simulink model "s_c_nbe_m32k"  (R2016b)
(part 2 of 104)

      mask prompts: io_dir "I/O direction"; io_delay "I/O delay"; init_val "Initial Value"; sample_period "Sample period"; names "Bitfield names [msb...lsb]"; bitwidths "Bitfield widths"; bin_pts "Bitfield binary pts"; arith_types "Bitfield types, ufix=0, fix=1, bool=2"; sim_port "Provide sim input/output?"; show_format "Print format string?"
      mask help: A 32-bit software-accessible register. Can be divided into bitfields of varying widths and types using the fields in the block mask.
      mask init:
      | swreg_init(gcb)
      settings: AttributesFormatString=1input:uf16.15 = 16 bits
      mask TypeOptions io_dir: To Processor | From Processor
      mask Callback io_dir:
      | mask_enables = get_param(gcb, 'MaskEnables');
      | mask_names = get_param(gcb, 'MaskNames');
      | if strcmp(get_param(gcb, 'io_dir'), 'To Processor'),
      |     mask_enables{ismember(mask_names, 'sample_period')} = 'off';
      | else
      |     mask_enables{ismember(mask_names, 'sample_period')} = 'on';
      | end
      | set_param(gcb, 'MaskEnables', mask_enables);
      mask DialogControl ParameterTabVar0 Prompt: Setup
  scale_p1_ddc0 : Subsystem  Tag=xps:sw_reg  AncestorBlock=xps_library/Memory/software_register  mask(swreg){io_dir=From Processor, io_delay=1, init_val=0, sample_period=1, names=scale, bitwidths=16, bin_pts=15, arith_types=0, sim_port=on, show_format=on}
      mask prompts: io_dir "I/O direction"; io_delay "I/O delay"; init_val "Initial Value"; sample_period "Sample period"; names "Bitfield names [msb...lsb]"; bitwidths "Bitfield widths"; bin_pts "Bitfield binary pts"; arith_types "Bitfield types, ufix=0, fix=1, bool=2"; sim_port "Provide sim input/output?"; show_format "Print format string?"
      mask help: A 32-bit software-accessible register. Can be divided into bitfields of varying widths and types using the fields in the block mask.
      mask init:
      | swreg_init(gcb)
      settings: AttributesFormatString=1input:uf16.15 = 16 bits
      mask TypeOptions io_dir: To Processor | From Processor
      mask Callback io_dir:
      | mask_enables = get_param(gcb, 'MaskEnables');
      | mask_names = get_param(gcb, 'MaskNames');
      | if strcmp(get_param(gcb, 'io_dir'), 'To Processor'),
      |     mask_enables{ismember(mask_names, 'sample_period')} = 'off';
      | else
      |     mask_enables{ismember(mask_names, 'sample_period')} = 'on';
      | end
      | set_param(gcb, 'MaskEnables', mask_enables);
      mask DialogControl ParameterTabVar0 Prompt: Setup
  sync_time_lsw : Subsystem  Tag=xps:sw_reg  AncestorBlock=xps_library/Memory/software_register  mask(swreg){io_dir=To Processor, io_delay=0, init_val=0, sample_period=1, names=reg, bitwidths=32, bin_pts=0, arith_types=0, sim_port=off, show_format=on}
      mask prompts: io_dir "I/O direction"; io_delay "I/O delay"; init_val "Initial Value"; sample_period "Sample period"; names "Bitfield names [msb...lsb]"; bitwidths "Bitfield widths"; bin_pts "Bitfield binary pts"; arith_types "Bitfield types, ufix=0, fix=1, bool=2"; sim_port "Provide sim input/output?"; show_format "Print format string?"
      mask help: A 32-bit software-accessible register. Can be divided into bitfields of varying widths and types using the fields in the block mask.
      mask init:
      | swreg_init(gcb)
      settings: AttributesFormatString=1output:uf32.0 = 32 bits
      mask TypeOptions io_dir: To Processor | From Processor
      mask Callback io_dir:
      | mask_enables = get_param(gcb, 'MaskEnables');
      | mask_names = get_param(gcb, 'MaskNames');
      | if strcmp(get_param(gcb, 'io_dir'), 'To Processor'),
      |     mask_enables{ismember(mask_names, 'sample_period')} = 'off';
      | else
      |     mask_enables{ismember(mask_names, 'sample_period')} = 'on';
      | end
      | set_param(gcb, 'MaskEnables', mask_enables);
      mask DialogControl ParameterTabVar0 Prompt: Setup
  sync_time_msw : Subsystem  Tag=xps:sw_reg  AncestorBlock=xps_library/Memory/software_register  mask(swreg){io_dir=To Processor, io_delay=0, init_val=0, sample_period=1, names=reg, bitwidths=16, bin_pts=0, arith_types=0, sim_port=off, show_format=on}
      mask prompts: io_dir "I/O direction"; io_delay "I/O delay"; init_val "Initial Value"; sample_period "Sample period"; names "Bitfield names [msb...lsb]"; bitwidths "Bitfield widths"; bin_pts "Bitfield binary pts"; arith_types "Bitfield types, ufix=0, fix=1, bool=2"; sim_port "Provide sim input/output?"; show_format "Print format string?"
      mask help: A 32-bit software-accessible register. Can be divided into bitfields of varying widths and types using the fields in the block mask.
      mask init:
      | swreg_init(gcb)
      settings: AttributesFormatString=1output:uf16.0 = 16 bits
      mask TypeOptions io_dir: To Processor | From Processor
      mask Callback io_dir:
      | mask_enables = get_param(gcb, 'MaskEnables');
      | mask_names = get_param(gcb, 'MaskNames');
      | if strcmp(get_param(gcb, 'io_dir'), 'To Processor'),
      |     mask_enables{ismember(mask_names, 'sample_period')} = 'off';
      | else
      |     mask_enables{ismember(mask_names, 'sample_period')} = 'on';
      | end
      | set_param(gcb, 'MaskEnables', mask_enables);
      mask DialogControl ParameterTabVar0 Prompt: Setup
  time_gen : Subsystem  mask{n_bits_period=fft_stages-1-2, n_bits_increment=0, n_bits_counter=48-fft_stages}
      mask prompts: n_bits_period "Period (2^?)"; n_bits_increment "Increment (2^?)"; n_bits_counter "Counter size (2^?)"
  time_gen1 : Subsystem  mask{n_bits_period=fft_stages-1-2-1+8, n_bits_increment=0, n_bits_counter=48-(fft_stages+8)}
      mask prompts: n_bits_period "Period (2^?)"; n_bits_increment "Increment (2^?)"; n_bits_counter "Counter size (2^?)"
  tl_cd0_control : Subsystem  Tag=xps:sw_reg  AncestorBlock=xps_library/Memory/software_register  mask(swreg){io_dir=From Processor, io_delay=0, init_val=0, sample_period=1, names=load_time_lsw, bitwidths=32, bin_pts=0, arith_types=0, sim_port=on, show_format=on}
      mask prompts: io_dir "I/O direction"; io_delay "I/O delay"; init_val "Initial Value"; sample_period "Sample period"; names "Bitfield names [msb...lsb]"; bitwidths "Bitfield widths"; bin_pts "Bitfield binary pts"; arith_types "Bitfield types, ufix=0, fix=1, bool=2"; sim_port "Provide sim input/output?"; show_format "Print format string?"
      mask help: A 32-bit software-accessible register. Can be divided into bitfields of varying widths and types using the fields in the block mask.
      mask init:
      | swreg_init(gcb)
      settings: AttributesFormatString=1input:uf32.0 = 32 bits
      mask TypeOptions io_dir: To Processor | From Processor
      mask Callback io_dir:
      | mask_enables = get_param(gcb, 'MaskEnables');
      | mask_names = get_param(gcb, 'MaskNames');
      | if strcmp(get_param(gcb, 'io_dir'), 'To Processor'),
      |     mask_enables{ismember(mask_names, 'sample_period')} = 'off';
      | else
      |     mask_enables{ismember(mask_names, 'sample_period')} = 'on';
      | end
      | set_param(gcb, 'MaskEnables', mask_enables);
      mask DialogControl ParameterTabVar0 Prompt: Setup
  tl_cd0_control0 : Subsystem  Tag=xps:sw_reg  AncestorBlock=xps_library/Memory/software_register  mask(swreg){io_dir=From Processor, io_delay=0, init_val=0, sample_period=1, names=[arm load_immediate load_time_msw], bitwidths=[1 1 16], bin_pts=[0 0 0], arith_types=[2 2 0], sim_port=on, show_format=on}
      mask prompts: io_dir "I/O direction"; io_delay "I/O delay"; init_val "Initial Value"; sample_period "Sample period"; names "Bitfield names [msb...lsb]"; bitwidths "Bitfield widths"; bin_pts "Bitfield binary pts"; arith_types "Bitfield types, ufix=0, fix=1, bool=2"; sim_port "Provide sim input/output?"; show_format "Print format string?"
      mask help: A 32-bit software-accessible register. Can be divided into bitfields of varying widths and types using the fields in the block mask.
      mask init:
      | swreg_init(gcb)
      settings: AttributesFormatString=3 inputs:b,b,uf16.0 = 18 bits
      mask TypeOptions io_dir: To Processor | From Processor
      mask Callback io_dir:
      | mask_enables = get_param(gcb, 'MaskEnables');
      | mask_names = get_param(gcb, 'MaskNames');
      | if strcmp(get_param(gcb, 'io_dir'), 'To Processor'),
      |     mask_enables{ismember(mask_names, 'sample_period')} = 'off';
      | else
      |     mask_enables{ismember(mask_names, 'sample_period')} = 'on';
      | end
      | set_param(gcb, 'MaskEnables', mask_enables);
      mask DialogControl ParameterTabVar0 Prompt: Setup
  tl_cd1_control : Subsystem  Tag=xps:sw_reg  AncestorBlock=xps_library/Memory/software_register  mask(swreg){io_dir=From Processor, io_delay=0, init_val=0, sample_period=1, names=load_time_lsw, bitwidths=32, bin_pts=0, arith_types=0, sim_port=on, show_format=on}
      mask prompts: io_dir "I/O direction"; io_delay "I/O delay"; init_val "Initial Value"; sample_period "Sample period"; names "Bitfield names [msb...lsb]"; bitwidths "Bitfield widths"; bin_pts "Bitfield binary pts"; arith_types "Bitfield types, ufix=0, fix=1, bool=2"; sim_port "Provide sim input/output?"; show_format "Print format string?"
      mask help: A 32-bit software-accessible register. Can be divided into bitfields of varying widths and types using the fields in the block mask.
      mask init:
      | swreg_init(gcb)
      settings: AttributesFormatString=1input:uf32.0 = 32 bits
      mask TypeOptions io_dir: To Processor | From Processor
      mask Callback io_dir:
      | mask_enables = get_param(gcb, 'MaskEnables');
      | mask_names = get_param(gcb, 'MaskNames');
      | if strcmp(get_param(gcb, 'io_dir'), 'To Processor'),
      |     mask_enables{ismember(mask_names, 'sample_period')} = 'off';
      | else
      |     mask_enables{ismember(mask_names, 'sample_period')} = 'on';
      | end
      | set_param(gcb, 'MaskEnables', mask_enables);
      mask DialogControl ParameterTabVar0 Prompt: Setup
  tl_cd1_control0 : Subsystem  Tag=xps:sw_reg  AncestorBlock=xps_library/Memory/software_register  mask(swreg){io_dir=From Processor, io_delay=0, init_val=0, sample_period=1, names=[arm load_immediate load_time_msw], bitwidths=[1 1 16], bin_pts=[0 0 0], arith_types=[2 2 0], sim_port=on, show_format=on}
      mask prompts: io_dir "I/O direction"; io_delay "I/O delay"; init_val "Initial Value"; sample_period "Sample period"; names "Bitfield names [msb...lsb]"; bitwidths "Bitfield widths"; bin_pts "Bitfield binary pts"; arith_types "Bitfield types, ufix=0, fix=1, bool=2"; sim_port "Provide sim input/output?"; show_format "Print format string?"
      mask help: A 32-bit software-accessible register. Can be divided into bitfields of varying widths and types using the fields in the block mask.
      mask init:
      | swreg_init(gcb)
      settings: AttributesFormatString=3 inputs:b,b,uf16.0 = 18 bits
      mask TypeOptions io_dir: To Processor | From Processor
      mask Callback io_dir:
      | mask_enables = get_param(gcb, 'MaskEnables');
      | mask_names = get_param(gcb, 'MaskNames');
      | if strcmp(get_param(gcb, 'io_dir'), 'To Processor'),
      |     mask_enables{ismember(mask_names, 'sample_period')} = 'off';
      | else
      |     mask_enables{ismember(mask_names, 'sample_period')} = 'on';
      | end
      | set_param(gcb, 'MaskEnables', mask_enables);
      mask DialogControl ParameterTabVar0 Prompt: Setup
  tl_fd0 : Subsystem  mask(timed_latch){n_bits_time=48-fft_stages, n_bits_quantization=fft_stages, n_bits_counters=4}
      mask prompts: n_bits_time "Number bits in time to compare"; n_bits_quantization "Time offset from lsb"; n_bits_counters "Bits in status counters"
      mask help:
      | Latches load_value when armed and current_time matches requested time.
      | current_time should be in ADC samples.
      mask init:
      | set_param([gcb,'/status'], 'bitwidths', mat2str([1, repmat(n_bits_counters, 1, 2)]));
      mask Help:
      | When armed, will latch new value when current time matches the time
      | specified. The input time should be in samples and mask settings allow
      | a portion of this to be compared to cater for quantization. Arm and latch
      | counts allow the current state, pending and missed latch events to be
      | determined.
  tl_fd1 : Subsystem  mask(timed_latch){n_bits_time=48-fft_stages, n_bits_quantization=fft_stages, n_bits_counters=4}
      mask prompts: n_bits_time "Number bits in time to compare"; n_bits_quantization "Time offset from lsb"; n_bits_counters "Bits in status counters"
      mask help:
      | Latches load_value when armed and current_time matches requested time.
      | current_time should be in ADC samples.
      mask init:
      | set_param([gcb,'/status'], 'bitwidths', mat2str([1, repmat(n_bits_counters, 1, 2)]));
      mask Help:
      | When armed, will latch new value when current time matches the time
      | specified. The input time should be in samples and mask settings allow
      | a portion of this to be compared to cater for quantization. Arm and latch
      | counts allow the current state, pending and missed latch events to be
      | determined.
  tvg : Subsystem
  tvg_tone_levels : Subsystem  Tag=xps:sw_reg  AncestorBlock=xps_library/Memory/software_register  mask(swreg){io_dir=From Processor, io_delay=0, init_val=0, sample_period=1, names=[p0r p0i p1r p1i], bitwidths=8, bin_pts=7, arith_types=1, sim_port=on, show_format=on}
      mask prompts: io_dir "I/O direction"; io_delay "I/O delay"; init_val "Initial Value"; sample_period "Sample period"; names "Bitfield names [msb...lsb]"; bitwidths "Bitfield widths"; bin_pts "Bitfield binary pts"; arith_types "Bitfield types, ufix=0, fix=1, bool=2"; sim_port "Provide sim input/output?"; show_format "Print format string?"
      mask help: A 32-bit software-accessible register. Can be divided into bitfields of varying widths and types using the fields in the block mask.
      mask init:
      | swreg_init(gcb)
      settings: AttributesFormatString=4 inputs:f8.7,f8.7,f8.7,f8.7 = 32 bits
      mask TypeOptions io_dir: To Processor | From Processor
      mask Callback io_dir:
      | mask_enables = get_param(gcb, 'MaskEnables');
      | mask_names = get_param(gcb, 'MaskNames');
      | if strcmp(get_param(gcb, 'io_dir'), 'To Processor'),
      |     mask_enables{ismember(mask_names, 'sample_period')} = 'off';
      | else
      |     mask_enables{ismember(mask_names, 'sample_period')} = 'on';
      | end
      | set_param(gcb, 'MaskEnables', mask_enables);
      mask DialogControl ParameterTabVar0 Prompt: Setup
  tvg_tone_targets : Subsystem  Tag=xps:sw_reg  AncestorBlock=xps_library/Memory/software_register  mask(swreg){io_dir=From Processor, io_delay=0, init_val=0, sample_period=1, names=[p0 p1], bitwidths=fft_stages, bin_pts=0, arith_types=0, sim_port=on, show_format=on}
      mask prompts: io_dir "I/O direction"; io_delay "I/O delay"; init_val "Initial Value"; sample_period "Sample period"; names "Bitfield names [msb...lsb]"; bitwidths "Bitfield widths"; bin_pts "Bitfield binary pts"; arith_types "Bitfield types, ufix=0, fix=1, bool=2"; sim_port "Provide sim input/output?"; show_format "Print format string?"
      mask help: A 32-bit software-accessible register. Can be divided into bitfields of varying widths and types using the fields in the block mask.
      mask init:
      | swreg_init(gcb)
      settings: AttributesFormatString=2 inputs:uf13.0,uf13.0 = 26 bits
      mask TypeOptions io_dir: To Processor | From Processor
      mask Callback io_dir:
      | mask_enables = get_param(gcb, 'MaskEnables');
      | mask_names = get_param(gcb, 'MaskNames');
      | if strcmp(get_param(gcb, 'io_dir'), 'To Processor'),
      |     mask_enables{ismember(mask_names, 'sample_period')} = 'off';
      | else
      |     mask_enables{ismember(mask_names, 'sample_period')} = 'on';
      | end
      | set_param(gcb, 'MaskEnables', mask_enables);
      mask DialogControl ParameterTabVar0 Prompt: Setup
  we_delay1 : Subsystem  AncestorBlock=casper_library_delays/pipeline  mask(pipeline){latency=2}
      mask help:
      | An explicitly laid-out delay line to avoid mapping to SRL16s
      | for use in pipelining to help achieve timing closure.
      mask init:
      | pipeline_init(gcb,'latency',latency);
      settings: AttributesFormatString=Latency = %<latency>
      mask Display:
      | port_label('input', 1, 'd');
      | port_label('output', 1, 'q');
      | disp(['Z^-', num2str(latency)]);
  we_delay112 : Subsystem  AncestorBlock=casper_library_delays/pipeline  mask(pipeline){latency=2}
      mask help:
      | An explicitly laid-out delay line to avoid mapping to SRL16s
      | for use in pipelining to help achieve timing closure.
      mask init:
      | pipeline_init(gcb,'latency',latency);
      settings: AttributesFormatString=Latency = %<latency>
      mask Display:
      | port_label('input', 1, 'd');
      | port_label('output', 1, 'q');
      | disp(['Z^-', num2str(latency)]);
  we_delay113 : Subsystem  AncestorBlock=casper_library_delays/pipeline  mask(pipeline){latency=2}
      mask help:
      | An explicitly laid-out delay line to avoid mapping to SRL16s
      | for use in pipelining to help achieve timing closure.
      mask init:
      | pipeline_init(gcb,'latency',latency);
      settings: AttributesFormatString=Latency = %<latency>
      mask Display:
      | port_label('input', 1, 'd');
      | port_label('output', 1, 'q');
      | disp(['Z^-', num2str(latency)]);
  we_delay114 : Subsystem  AncestorBlock=casper_library_delays/pipeline  mask(pipeline){latency=2}
      mask help:
      | An explicitly laid-out delay line to avoid mapping to SRL16s
      | for use in pipelining to help achieve timing closure.
      mask init:
      | pipeline_init(gcb,'latency',latency);
      settings: AttributesFormatString=Latency = %<latency>
      mask Display:
      | port_label('input', 1, 'd');
      | port_label('output', 1, 'q');
      | disp(['Z^-', num2str(latency)]);
  we_delay115 : Subsystem  AncestorBlock=casper_library_delays/pipeline  mask(pipeline){latency=2}
      mask help:
      | An explicitly laid-out delay line to avoid mapping to SRL16s
      | for use in pipelining to help achieve timing closure.
      mask init:
      | pipeline_init(gcb,'latency',latency);
      settings: AttributesFormatString=Latency = %<latency>
      mask Display:
      | port_label('input', 1, 'd');
      | port_label('output', 1, 'q');
      | disp(['Z^-', num2str(latency)]);
  we_delay116 : Subsystem  AncestorBlock=casper_library_delays/pipeline  mask(pipeline){latency=2}
      mask help:
      | An explicitly laid-out delay line to avoid mapping to SRL16s
      | for use in pipelining to help achieve timing closure.
      mask init:
      | pipeline_init(gcb,'latency',latency);
      settings: AttributesFormatString=Latency = %<latency>
      mask Display:
      | port_label('input', 1, 'd');
      | port_label('output', 1, 'q');
      | disp(['Z^-', num2str(latency)]);
  we_delay117 : Subsystem  AncestorBlock=casper_library_delays/pipeline  mask(pipeline){latency=2}
      mask help:
      | An explicitly laid-out delay line to avoid mapping to SRL16s
      | for use in pipelining to help achieve timing closure.
      mask init:
      | pipeline_init(gcb,'latency',latency);
      settings: AttributesFormatString=Latency = %<latency>
      mask Display:
      | port_label('input', 1, 'd');
      | port_label('output', 1, 'q');
      | disp(['Z^-', num2str(latency)]);
  we_delay124 : Subsystem  AncestorBlock=casper_library_delays/pipeline  mask(pipeline){latency=2}
      mask help:
      | An explicitly laid-out delay line to avoid mapping to SRL16s
      | for use in pipelining to help achieve timing closure.
      mask init:
      | pipeline_init(gcb,'latency',latency);
      settings: AttributesFormatString=Latency = %<latency>
      mask Display:
      | port_label('input', 1, 'd');
      | port_label('output', 1, 'q');
      | disp(['Z^-', num2str(latency)]);
  we_delay126 : Subsystem  AncestorBlock=casper_library_delays/pipeline  mask(pipeline){latency=2}
      mask help:
      | An explicitly laid-out delay line to avoid mapping to SRL16s
      | for use in pipelining to help achieve timing closure.
      mask init:
      | pipeline_init(gcb,'latency',latency);
      settings: AttributesFormatString=Latency = %<latency>
      mask Display:
      | port_label('input', 1, 'd');
      | port_label('output', 1, 'q');
      | disp(['Z^-', num2str(latency)]);
  we_delay13 : Subsystem  AncestorBlock=casper_library_delays/pipeline  mask(pipeline){latency=2}
      mask help:
      | An explicitly laid-out delay line to avoid mapping to SRL16s
      | for use in pipelining to help achieve timing closure.
      mask init:
      | pipeline_init(gcb,'latency',latency);
      settings: AttributesFormatString=Latency = %<latency>
      mask Display:
      | port_label('input', 1, 'd');
      | port_label('output', 1, 'q');
      | disp(['Z^-', num2str(latency)]);
  we_delay2 : Subsystem  AncestorBlock=casper_library_delays/pipeline  mask(pipeline){latency=2}
      mask help:
      | An explicitly laid-out delay line to avoid mapping to SRL16s
      | for use in pipelining to help achieve timing closure.
      mask init:
      | pipeline_init(gcb,'latency',latency);
      settings: AttributesFormatString=Latency = %<latency>
      mask Display:
      | port_label('input', 1, 'd');
      | port_label('output', 1, 'q');
      | disp(['Z^-', num2str(latency)]);
  we_delay29 : Subsystem  AncestorBlock=casper_library_delays/pipeline  mask(pipeline){latency=2}
      mask help:
      | An explicitly laid-out delay line to avoid mapping to SRL16s
      | for use in pipelining to help achieve timing closure.
      mask init:
      | pipeline_init(gcb,'latency',latency);
      settings: AttributesFormatString=Latency = %<latency>
      mask Display:
      | port_label('input', 1, 'd');
      | port_label('output', 1, 'q');
      | disp(['Z^-', num2str(latency)]);
  we_delay37 : Subsystem  AncestorBlock=casper_library_delays/pipeline  mask(pipeline){latency=2}
      mask help:
      | An explicitly laid-out delay line to avoid mapping to SRL16s
      | for use in pipelining to help achieve timing closure.
      mask init:
      | pipeline_init(gcb,'latency',latency);
      settings: AttributesFormatString=Latency = %<latency>
      mask Display:
      | port_label('input', 1, 'd');
      | port_label('output', 1, 'q');
      | disp(['Z^-', num2str(latency)]);
  we_delay38 : Subsystem  AncestorBlock=casper_library_delays/pipeline  mask(pipeline){latency=2}
      mask help:
      | An explicitly laid-out delay line to avoid mapping to SRL16s
      | for use in pipelining to help achieve timing closure.
      mask init:
      | pipeline_init(gcb,'latency',latency);
      settings: AttributesFormatString=Latency = %<latency>
      mask Display:
      | port_label('input', 1, 'd');
      | port_label('output', 1, 'q');
      | disp(['Z^-', num2str(latency)]);
  we_delay39 : Subsystem  AncestorBlock=casper_library_delays/pipeline  mask(pipeline){latency=2}
      mask help:
      | An explicitly laid-out delay line to avoid mapping to SRL16s
      | for use in pipelining to help achieve timing closure.
      mask init:
      | pipeline_init(gcb,'latency',latency);
      settings: AttributesFormatString=Latency = %<latency>
      mask Display:
      | port_label('input', 1, 'd');
      | port_label('output', 1, 'q');
      | disp(['Z^-', num2str(latency)]);
  we_delay41 : Subsystem  AncestorBlock=casper_library_delays/pipeline  mask(pipeline){latency=2}
      mask help:
      | An explicitly laid-out delay line to avoid mapping to SRL16s
      | for use in pipelining to help achieve timing closure.
      mask init:
      | pipeline_init(gcb,'latency',latency);
      settings: AttributesFormatString=Latency = %<latency>
      mask Display:
      | port_label('input', 1, 'd');
      | port_label('output', 1, 'q');
      | disp(['Z^-', num2str(latency)]);
  we_delay47 : Subsystem  AncestorBlock=casper_library_delays/pipeline  mask(pipeline){latency=2}
      mask help:
      | An explicitly laid-out delay line to avoid mapping to SRL16s
      | for use in pipelining to help achieve timing closure.
      mask init:
      | pipeline_init(gcb,'latency',latency);
      settings: AttributesFormatString=Latency = %<latency>
      mask Display:
      | port_label('input', 1, 'd');
      | port_label('output', 1, 'q');
      | disp(['Z^-', num2str(latency)]);
  we_delay48 : Subsystem  AncestorBlock=casper_library_delays/pipeline  mask(pipeline){latency=2}
      mask help:
      | An explicitly laid-out delay line to avoid mapping to SRL16s
      | for use in pipelining to help achieve timing closure.
      mask init:
      | pipeline_init(gcb,'latency',latency);
      settings: AttributesFormatString=Latency = %<latency>
      mask Display:
      | port_label('input', 1, 'd');
      | port_label('output', 1, 'q');
      | disp(['Z^-', num2str(latency)]);
  we_delay49 : Subsystem  AncestorBlock=casper_library_delays/pipeline  mask(pipeline){latency=2}
      mask help:
      | An explicitly laid-out delay line to avoid mapping to SRL16s
      | for use in pipelining to help achieve timing closure.
      mask init:
      | pipeline_init(gcb,'latency',latency);
      settings: AttributesFormatString=Latency = %<latency>
      mask Display:
      | port_label('input', 1, 'd');
      | port_label('output', 1, 'q');
      | disp(['Z^-', num2str(latency)]);
  we_delay50 : Subsystem  AncestorBlock=casper_library_delays/pipeline  mask(pipeline){latency=2}
      mask help:
      | An explicitly laid-out delay line to avoid mapping to SRL16s
      | for use in pipelining to help achieve timing closure.
      mask init:
      | pipeline_init(gcb,'latency',latency);
      settings: AttributesFormatString=Latency = %<latency>
      mask Display:
      | port_label('input', 1, 'd');
      | port_label('output', 1, 'q');
      | disp(['Z^-', num2str(latency)]);
  we_delay7 : Subsystem  AncestorBlock=casper_library_delays/pipeline  mask(pipeline){latency=2}
      mask help:
      | An explicitly laid-out delay line to avoid mapping to SRL16s
      | for use in pipelining to help achieve timing closure.
      mask init:
      | pipeline_init(gcb,'latency',latency);
      settings: AttributesFormatString=Latency = %<latency>
      mask Display:
      | port_label('input', 1, 'd');
      | port_label('output', 1, 'q');
      | disp(['Z^-', num2str(latency)]);
  tag scope: cnt_rst=global, ct_board_hmc_offset=global, ct_chans_per_board=global, ct_chans_per_x=global, ct_chans_per_x_hmc_par=global, ct_chans_per_x_hmc_par_recip=global, ct_chans_per_x_par=global, ct_chans_per_x_recip=global, ct_fake_data_error=global, ct_freq_gen_offset=global, ct_num_x_boards=global, ct_num_x_boards_recip=global, ct_num_xeng=global, ct_num_xeng_recip=global, ct_rst_err_latch=global, ct_tag_insert_sel=global, ct_tvg_en2=global, ct_tvg_en=global, ct_x_per_board=global, ct_x_per_board_recip=global, force_gbe_txen=global, local_time_capture=global, local_time_src=global, obuf_read_gap=global, pfb_bypass=global, snap_reord_mux_we_sel=global, snap_stop_mux_sel=global, sys_rst=global, ts_tvg_en=global, tvgtone_levels=global, tvgtone_p0=global, tvgtone_p1=global
  wires:
  cwg0/1(bus_out) -> pipeline9/1(d), pipeline95/1(d)
  cwg0/3(rpt_rst) -> Terminator61/1
  pipeline95/1(q) -> [cwg0]
  Constant2/1 -> [mrst]
  edge_detect1/1(out) -> pipeline11/1(d)
  pipeline9/1(q) -> [cwg1]
  pipeline11/1(q) -> [sync]
  cwg0/2(dvalid) -> Terminator3/1
  Constant11/1 -> Delay14/1
  Delay14/1 -> pipeline10/1(d), edge_detect1/1(in)
  pipeline10/1(q) -> [dvalid]
  pipeline13/1(q) -> [osc_cos_ddc0]
  cwg1/1(bus_out) -> pipeline13/1(d)
  cwg1/3(rpt_rst) -> Terminator65/1
  cwg1/2(dvalid) -> Terminator1/1
  Gateway Out7/1 -> To Workspace12/1
  Gateway Out1/1 -> To Workspace3/1
  Gateway Out3/1 -> To Workspace11/1
  Gateway Out6/1 -> To Workspace10/1
  bus_expand1/1(msb_out8) -> Gateway Out1/1
  bus_expand1/2(out7) -> Gateway Out7/1
  bus_expand1/4(out5) -> Gateway Out6/1
  bus_expand1/3(out6) -> Gateway Out3/1
  bus_expand1/8(lsb_out1) -> Gateway Out10/1
  bus_expand1/7(out2) -> Gateway Out9/1
  bus_expand1/6(out3) -> Gateway Out11/1
  bus_expand1/5(out4) -> Gateway Out8/1
  Gateway Out10/1 -> To Workspace6/1
  Gateway Out9/1 -> To Workspace7/1
  Gateway Out11/1 -> To Workspace8/1
  Gateway Out8/1 -> To Workspace9/1
  [cwg0] -> bus_expand1/1(bus_in)
  Constant57/1 -> scale_p0_ddc0/1(sim_1)
  Constant1/1 -> scale_p1_ddc0/1(sim_1)
  [sync] -> DDC/1(sync)
  [dvalid] -> DDC/2(dvalid)
  [cwg0] -> DDC/3(pol0_data)
  [osc_cos_ddc0] -> DDC/4(osc0)
  scale_p0_ddc0/1(in_scale) -> DDC/5(scale0)
  [cwg1] -> DDC/6(pol1_data)
  [osc_cos_ddc0] -> DDC/7(osc1)
  scale_p1_ddc0/1(in_scale) -> DDC/8(scale1)
  DDC/1(sync_out) -> [ddc_sync]
  DDC/2(pol0_ddc) -> [ddc_pol0]
  DDC/3(pol1_ddc) -> [ddc_pol1]
  DDC/4(dvalid_out) -> [ddc_dvalid]
  Gateway Out65/1 -> To Workspace69/1
  [ddc_dvalid] -> Gateway Out65/1
  Gateway Out4/1 -> To Workspace1/1
  [ddc_pol1] -> Gateway Out4/1
  edge_detect5/1(out) -> pipeline15/1(d)
  control/7(in_cnt_rst) -> edge_detect3/1(in)
  edge_detect3/1(out) -> pipeline14/1(d)
  control/3(in_gbe_rst) -> pipeline17/1(d)
  control/1(in_sys_rst) -> pipeline8/1(d)
  pipeline8/1(q) -> [sys_rst]
  pipeline15/1(q) -> [clr_status]
  pipeline17/1(q) -> [gbe_rst]
  pipeline18/1(q) -> [gbe_txen]
  pipeline6/1(q) -> [tvg_adc0_en]
  pipeline14/1(q) -> [cnt_rst]
  control/5(in_tvg_adc0) -> pipeline6/1(d)
  edge_detect4/1(out) -> pipeline38/1(d)
  pipeline38/1(q) -> [gbe_cnt_rst]
  control/8(in_gbe_cnt_rst) -> edge_detect4/1(in)
  control/4(in_gbe_txen) -> pipeline18/1(d)
  control/2(in_status_clr) -> edge_detect5/1(in)
  pipeline43/1(q) -> [adc_snap_arm]
  control/9(in_adc_snap_arm) -> pipeline43/1(d)
  control/10(in_adc_snap_trig_select) -> pipeline39/1(d)
  pipeline39/1(q) -> [adc_snap_trig_source]
  pipeline59/1(q) -> [ct_tvg_en]
  control/11(in_ct_tvg_en) -> pipeline59/1(d)
  pipeline52/1(q) -> [up_dbg_rst]
  control/12(in_unpack_debug_reset) -> pipeline52/1(d)
  control/13(in_cd_bypass) -> pipeline131/1(d)
  pipeline131/1(q) -> [cd_bypass]
  pipeline93/1(q) -> [tvg_adc1_en]
  control/6(in_tvg_adc1) -> pipeline93/1(d)
  control/14(in_gbe_stopmux) -> pipeline19/1(d)
  pipeline19/1(q) -> [gbe_stopmux]
  control/15(in_pfb_bypass) -> pipeline66/1(d)
  pipeline66/1(q) -> [pfb_bypass]
  control/16(in_ts_tvg_en) -> pipeline148/1(d)
  pipeline148/1(q) -> [ts_tvg_en]
  control/17(in_force_gbe_txen) -> pipeline7/1(d)
  pipeline7/1(q) -> [force_gbe_txen]
  control/18(in_snap_stop_mux_sel) -> pipeline127/1(d)
  control/19(in_snap_reord_mux_we_sel) -> pipeline128/1(d)
  pipeline127/1(q) -> [snap_stop_mux_sel]
  pipeline128/1(q) -> [snap_reord_mux_we_sel]
  control/20(in_local_time_source) -> pipeline5/1(d)
  edge_detect6/1(out) -> pipeline164/1(d)
  pipeline164/1(q) -> [local_time_capture]
  pipeline5/1(q) -> [local_time_src]
  control/21(in_local_time_capture) -> edge_detect6/1(in)
  control/22(in_time_diff_check_en) -> pipeline47/1(d)
  pipeline47/1(q) -> [time_diff_check_en]
  control/23(in_auto_rst_enable) -> pipeline132/1(d)
  pipeline132/1(q) -> [auto_rst_enable]
  [ddc_sync] -> nb_pfb/1(sync)
  [ddc_pol0] -> nb_pfb/2(pol0)
  [ddc_pol1] -> nb_pfb/3(pol1)
  [ddc_dvalid] -> nb_pfb/4(dvalid)
  nb_pfb/1(sync_out) -> [pfb_sync]
  nb_pfb/2(pol0_out) -> [pfb_d144_0]
  nb_pfb/3(pol1_out) -> [pfb_d144_1]
  nb_pfb/4(dvalid_out) -> [pfb_dv]
  Gateway Out2/1 -> To Workspace2/1
  [ddc_pol0] -> Gateway Out2/1
  Constant64/1 -> freq_cwg0/1(sim_1)
  scale_cwg0/1(in_scale) -> pipeline48/1(d)
  freq_cwg0/1(in_frequency) -> pipeline49/1(d)
  pipeline49/1(q) -> cwg0/1(freq)
  pipeline48/1(q) -> cwg0/2(scale)
  [mrst] -> pipeline180/1(d)
  Constant62/1 -> rpt_length_cwg0/1(sim_1)
  rpt_en_cwg0/1(in_en) -> Convert25/1
  Constant70/1 -> rpt_en_cwg0/1(sim_1)
  Convert25/1 -> pipeline181/1(d)
  rpt_length_cwg0/1(in_repeat_length) -> pipeline182/1(d)
  pipeline180/1(q) -> cwg0/3(rst)
  pipeline181/1(q) -> cwg0/4(repeat_en)
  pipeline182/1(q) -> cwg0/5(repeat_length)
  Constant106/1 -> cwg0/6(en)
  Constant37/1 -> scale_cwg0/1(sim_1)
  Constant79/1 -> freq_cwg_corr/1(sim_1)
  Constant80/1 -> scale_cwg_corr/1(sim_1)
  freq_cwg_corr/1(in_frequency) -> pipeline2/1(d)
  scale_cwg_corr/1(in_scale) -> pipeline1/1(d)
  pipeline147/1(q) -> cwg1/3(rst)
  rpt_en_cwg_corr/1(in_en) -> pipeline3/1(d)
  rpt_length_cwg_corr/1(in_repeat_length) -> pipeline12/1(d)
  Constant96/1 -> cwg1/6(en)
  [mrst] -> pipeline147/1(d)
  Constant97/1 -> rpt_en_cwg_corr/1(sim_1)
  Constant99/1 -> rpt_length_cwg_corr/1(sim_1)
  pipeline1/1(q) -> cwg1/2(scale)
  pipeline2/1(q) -> cwg1/1(freq)
  pipeline3/1(q) -> cwg1/4(repeat_en)
  pipeline12/1(q) -> cwg1/5(repeat_length)
  Gateway Out5/1 -> To Workspace4/1
  [dvalid] -> Gateway Out5/1
  [pfb_d144_0] -> bus_expand5/1(bus_in)
  Gateway Out12/1 -> To Workspace5/1
  bus_expand5/1(msb_out8) -> Gateway Out12/1
  Gateway Out13/1 -> To Workspace14/1
  Gateway Out14/1 -> To Workspace15/1
  Gateway Out15/1 -> To Workspace16/1
  bus_expand5/7(out2) -> Gateway Out15/1
  bus_expand5/5(out4) -> Gateway Out14/1
  bus_expand5/3(out6) -> Gateway Out13/1
  bus_expand5/2(out7) -> Gateway Out16/1
  bus_expand5/4(out5) -> Gateway Out17/1
  bus_expand5/6(out3) -> Gateway Out18/1
  bus_expand5/8(lsb_out1) -> Gateway Out19/1
  Gateway Out17/1 -> To Workspace17/1
  Gateway Out18/1 -> To Workspace18/1
  Gateway Out19/1 -> To Workspace19/1
  Gateway Out16/1 -> To Workspace13/1
  Gateway Out20/1 -> To Workspace20/1
  [pfb_sync] -> Gateway Out20/1
  Gateway Out21/1 -> To Workspace21/1
  [pfb_dv] -> Gateway Out21/1
  Concat22/1 -> [ld_val0]
  Concat3/1 -> [ld_val1]
  phase0/1(in_initial) -> Reinterpret2/1
  delta_delay0/1(in_delta) -> Reinterpret1/1
  phase0/2(in_delta) -> Reinterpret3/1
  Reinterpret8/1 -> Concat22/1
  Reinterpret1/1 -> Concat22/2
  Reinterpret2/1 -> Concat22/3
  Reinterpret3/1 -> Concat22/4
  phase1/1(in_initial) -> Reinterpret5/1
  delta_delay1/1(in_delta) -> Reinterpret4/1
  phase1/2(in_delta) -> Reinterpret6/1
  Reinterpret4/1 -> Concat3/2
  Reinterpret5/1 -> Concat3/3
  Reinterpret6/1 -> Concat3/4
  Reinterpret7/1 -> Concat3/1
  delay0/1(in_initial) -> Reinterpret8/1
  delay1/1(in_initial) -> Reinterpret7/1
  tl_cd0_control0/3(in_load_time_msw) -> Concat6/1
  tl_cd0_control/1(in_load_time_lsw) -> Concat6/2
  Constant42/1 -> tl_cd0_control/1(sim_1)
  Constant40/1 -> tl_cd0_control0/3(sim_3)
  Constant41/1 -> tl_cd0_control0/2(sim_2)
  Constant43/1 -> Delay12/1
  Delay12/1 -> tl_cd0_control0/1(sim_1)
  Concat6/1 -> pipeline136/1(d)
  tl_cd0_control0/2(in_load_immediate) -> pipeline135/1(d)
  tl_cd0_control0/1(in_arm) -> pipeline134/1(d)
  tl_cd1_control0/3(in_load_time_msw) -> Concat8/1
  tl_cd1_control/1(in_load_time_lsw) -> Concat8/2
  Constant47/1 -> tl_cd1_control/1(sim_1)
  Constant45/1 -> tl_cd1_control0/3(sim_3)
  Constant46/1 -> tl_cd1_control0/2(sim_2)
  Constant48/1 -> Delay13/1
  Delay13/1 -> tl_cd1_control0/1(sim_1)
  Concat8/1 -> pipeline143/1(d)
  tl_cd1_control0/2(in_load_immediate) -> pipeline138/1(d)
  tl_cd1_control0/1(in_arm) -> pipeline137/1(d)
  pipeline134/1(q) -> [tl_cd0_arm]
  pipeline135/1(q) -> [tl_cd0_load_immediate]
  pipeline136/1(q) -> [tl_cd0_load_time]
  pipeline138/1(q) -> [tl_cd1_load_immediate]
  pipeline137/1(q) -> [tl_cd1_arm]
  pipeline143/1(q) -> [tl_cd1_load_time]
  Counter2/1 -> pipeline29/1(d)
  Constant26/1 -> eq1/2(data_in)
  Constant4/1 -> eq1/3(we)
  Delay53/1 -> quant1/1(sync_in)
  Delay34/1 -> quant1/2(din)
  eq1/1(data_out) -> quant1/4(coeffs)
  Delay50/1 -> quant1/3(en)
  Counter4/1 -> pipeline27/1(d)
  Constant24/1 -> eq0/2(data_in)
  Constant25/1 -> eq0/3(we)
  Delay51/1 -> quant0/1(sync_in)
  Delay3/1 -> quant0/2(din)
  Delay52/1 -> quant0/3(en)
  eq0/1(data_out) -> quant0/4(coeffs)
  quant0/1(sync_out) -> [q_sync]
  quant0/2(dout) -> [q_d64_0]
  quant0/3(dvalid) -> [q_dv]
  quant0/4(of) -> [q_of0]
  quant1/2(dout) -> [q_d64_1]
  quant1/1(sync_out) -> Terminator19/1
  quant1/3(dvalid) -> Terminator21/1
  quant1/4(of) -> [q_of1]
  pipeline27/1(q) -> eq0/1(addr)
  pipeline29/1(q) -> eq1/1(addr)
  [fdfs_sync] -> Delay51/1, pipeline42/1(d)
  [fdfs_d144_0] -> Delay3/1
  [fdfs_dv] -> Delay52/1, pipeline41/1(d)
  pipeline41/1(q) -> Counter4/2
  pipeline42/1(q) -> Counter4/1
  pipeline45/1(q) -> Counter2/2
  [fdfs_sync] -> Delay53/1, pipeline4/1(d)
  [fdfs_d144_1] -> Delay34/1
  [fdfs_dv] -> Delay50/1, pipeline45/1(d)
  pipeline4/1(q) -> Counter2/1
  [clr_status] -> Subsystem5/1(rst)
  Subsystem5/1(out0) -> quant_status/1(out_pol0_or_cnt)
  Relational2/1 -> Subsystem5/2(in0)
  Constant10/1 -> Relational2/2
  [q_of0] -> Relational2/1
  Relational3/1 -> Subsystem5/3(in1)
  [q_of1] -> Relational3/1
  Constant13/1 -> Relational3/2
  Subsystem5/2(out1) -> quant_status/2(out_pol1_or_cnt)
  tl_fd0/2(enable) -> phase_compensation0/5(load_value)
  tl_fd1/1(value) -> phase_compensation1/4(delay_value)
  tl_fd1/2(enable) -> phase_compensation1/5(load_value)
  tl_fd0/1(value) -> phase_compensation0/4(delay_value)
  [clr_status] -> tl_fd0/1(rst), tl_fd1/1(rst)
  phase_compensation0/1(sync_out) -> [fdfs_sync]
  phase_compensation1/1(sync_out) -> Terminator24/1
  phase_compensation0/2(dout) -> [fdfs_d144_0]
  phase_compensation1/2(dout) -> [fdfs_d144_1]
  phase_compensation0/3(dvalid) -> [fdfs_dv]
  phase_compensation1/3(dvalid) -> Terminator25/1
  [ld_val0] -> tl_fd0/3(load_value)
  [ld_val1] -> tl_fd1/3(load_value)
  bus_expand16/1(msb_out2) -> tl_fd0/5(din)
  tl_fd0/5(dvalid) -> phase_compensation0/3(en)
  tl_fd0/3(sync_out) -> phase_compensation0/1(sync_in)
  tl_fd0/4(dout) -> phase_compensation0/2(din)
  tl_fd1/4(dout) -> phase_compensation1/2(din)
  bus_expand16/2(lsb_out1) -> tl_fd1/5(din)
  Constant29/1 -> Concat2/2
  Concat2/1 -> tl_fd1/2(current_time), [pfb_time], tl_fd0/2(current_time)
  tl_fd0/7(misco) -> Terminator2/1
  tl_fd0/6(time) -> Terminator4/1
  tl_fd1/6(time) -> Terminator5/1
  tl_fd1/3(sync_out) -> phase_compensation1/1(sync_in)
  tl_fd1/5(dvalid) -> phase_compensation1/3(en)
  tl_fd1/7(misco) -> Terminator6/1
  Constant18/1 -> tl_fd0/7(misci)
  Constant19/1 -> tl_fd1/7(misci)
  time_gen/1(rd_sync_out) -> tl_fd0/4(sync_in), tl_fd1/4(sync_in)
  time_gen/2(rd_dvalid) -> tl_fd1/6(en), tl_fd0/6(en)
  time_gen/3(rd_val_out) -> Concat2/1
  time_gen/4(rd_misc_out) -> bus_expand16/1(bus_in)
  [sync80] -> time_gen/1(wr_sync_in)
  [valid80] -> time_gen/2(wr_en)
  [pfb_sync] -> time_gen/4(rd_sync_in)
  [pfb_dv] -> time_gen/5(rd_en)
  [pfb_d144_1] -> Concat1/2
  [pfb_d144_0] -> Concat1/1
  Concat1/1 -> time_gen/6(rd_misc_in)
  [time80] -> time_gen/3(wr_val_in)
  [tl_cd0_load_time] -> tl_fd0/10(load_time)
  [tl_cd0_arm] -> tl_fd0/8(arm)
  [tl_cd0_load_immediate] -> tl_fd0/9(load_immediate)
  [tl_cd1_arm] -> tl_fd1/8(arm)
  [tl_cd1_load_immediate] -> tl_fd1/9(load_immediate)
  [tl_cd1_load_time] -> tl_fd1/10(load_time)
  Constant5/1 -> [sync80]
  Constant6/1 -> [valid80]
  Constant7/1 -> [time80]
  Gateway Out28/1 -> To Workspace27/1
  [q_of1] -> Gateway Out28/1
  Gateway Out29/1 -> To Workspace28/1
  [q_of0] -> Gateway Out29/1
  Gateway Out30/1 -> To Workspace29/1
  [q_dv] -> Gateway Out30/1
  Gateway Out31/1 -> To Workspace30/1
  [q_sync] -> Gateway Out31/1
  Gateway Out34/1 -> To Workspace33/1
  Gateway Out36/1 -> To Workspace34/1
  Gateway Out38/1 -> To Workspace35/1
  Gateway Out33/1 -> To Workspace32/1
  Gateway Out35/1 -> To Workspace36/1
  Gateway Out37/1 -> To Workspace37/1
  Gateway Out39/1 -> To Workspace38/1
  Gateway Out32/1 -> To Workspace31/1
  bus_expand3/1(msb_out8) -> Gateway Out32/1
  bus_expand3/2(out7) -> Gateway Out33/1
  bus_expand3/3(out6) -> Gateway Out34/1
  bus_expand3/4(out5) -> Gateway Out35/1
  bus_expand3/6(out3) -> Gateway Out37/1
  bus_expand3/5(out4) -> Gateway Out36/1
  bus_expand3/7(out2) -> Gateway Out38/1
  bus_expand3/8(lsb_out1) -> Gateway Out39/1
  [q_d64_0] -> bus_expand3/1(bus_in)
  [q_d64_1] -> bus_expand6/1(bus_in)
  bus_expand6/1(msb_out8) -> Gateway Out40/1
  bus_expand6/2(out7) -> Gateway Out42/1
  bus_expand6/3(out6) -> Gateway Out43/1
  bus_expand6/4(out5) -> Gateway Out44/1
  bus_expand6/6(out3) -> Gateway Out58/1
  bus_expand6/5(out4) -> Gateway Out51/1
  bus_expand6/7(out2) -> Gateway Out59/1
  bus_expand6/8(lsb_out1) -> Gateway Out60/1
  Gateway Out40/1 -> To Workspace39/1
  Gateway Out43/1 -> To Workspace42/1
  Gateway Out51/1 -> To Workspace43/1
  Gateway Out59/1 -> To Workspace44/1
  Gateway Out42/1 -> To Workspace40/1
  Gateway Out44/1 -> To Workspace52/1
  Gateway Out58/1 -> To Workspace53/1
  Gateway Out60/1 -> To Workspace55/1
  bus_expand2/1(msb_out8) -> Gateway Out22/1
  Gateway Out23/1 -> To Workspace23/1
  Gateway Out24/1 -> To Workspace25/1
  Gateway Out25/1 -> To Workspace26/1
  bus_expand2/7(out2) -> Gateway Out25/1
  bus_expand2/5(out4) -> Gateway Out24/1
  bus_expand2/3(out6) -> Gateway Out23/1
  bus_expand2/2(out7) -> Gateway Out26/1
  bus_expand2/4(out5) -> Gateway Out27/1
  bus_expand2/6(out3) -> Gateway Out41/1
  bus_expand2/8(lsb_out1) -> Gateway Out45/1
  Gateway Out27/1 -> To Workspace45/1
  Gateway Out41/1 -> To Workspace48/1
  Gateway Out45/1 -> To Workspace49/1
  Gateway Out26/1 -> To Workspace24/1
  Gateway Out46/1 -> To Workspace46/1
  [fdfs_sync] -> Gateway Out46/1
  Gateway Out47/1 -> To Workspace47/1
  [fdfs_dv] -> Gateway Out47/1
  Gateway Out22/1 -> To Workspace22/1
  [fdfs_d144_0] -> bus_expand2/1(bus_in)
  tvg_tone_levels/2(in_p0i) -> bus_create/2(in2)
  tvg_tone_levels/3(in_p1r) -> bus_create/3(in3)
  tvg_tone_levels/4(in_p1i) -> bus_create/4(in4)
  tvg_tone_levels/1(in_p0r) -> bus_create/1(in1)
  tvg_tone_targets/1(in_p0) -> Slice18/1
  tvg_tone_targets/2(in_p1) -> Slice19/1
  Constant51/1 -> tvg_tone_targets/1(sim_1)
  Constant52/1 -> tvg_tone_targets/2(sim_2)
  Constant8/1 -> tvg_tone_levels/4(sim_4)
  Constant3/1 -> tvg_tone_levels/1(sim_1)
  Constant27/1 -> tvg_tone_levels/3(sim_3)
  Constant9/1 -> tvg_tone_levels/2(sim_2)
  bus_create/1(bus_out) -> [tvgtone_levels]
  pipeline20/1(q) -> [outfreq_stopmux]
  ct_debug/6(in_outfreq_stopmux) -> pipeline20/1(d)
  pipeline21/1(q) -> [out_stopmux]
  ct_debug/5(in_out_stopmux) -> pipeline21/1(d)
  pipeline55/1(q) -> [wrrd_stopmux]
  ct_debug/3(in_wrrd_stopmux) -> pipeline55/1(d)
  pipeline56/1(q) -> [in_stopmux]
  ct_debug/1(in_in_stopmux) -> pipeline56/1(d)
  pipeline122/1(q) -> [ct_snap_arm]
  pipeline16/1(q) -> edge_detect7/1(in)
  ct_debug/8(in_snap_trig) -> pipeline16/1(d)
  ct_debug/7(in_snap_arm) -> pipeline122/1(d)
  edge_detect7/1(out) -> [ct_snap_trig]
  ct_debug/2(in_in_trigmux) -> pipeline150/1(d)
  pipeline150/1(q) -> [in_trigmux]
  ct_debug/4(in_obuf_stopmux) -> pipeline167/1(d)
  pipeline167/1(q) -> [obuf_stopmux]
  ct_debug/9(in_snap_wesel) -> pipeline22/1(d)
  pipeline22/1(q) -> [ct_snap_wesel]
  pipeline157/1(q) -> [ct_snap_trigsel]
  ct_debug/10(in_snap_trigsel) -> pipeline157/1(d)
  pipeline166/1(q) -> [ct_snap_circsel]
  ct_debug/11(in_snap_circsel) -> pipeline166/1(d)
  [ct_dv] -> Subsystem8/1(In1)
  Subsystem8/1(Out1) -> ct_out_dv_rate/1(out_reg)
  [cnt_rst] -> Subsystem10/1(rst)
  [obuf_ct_addr_err_g] -> Subsystem10/2(in0)
  [ct_sync] -> Subsystem10/3(in1)
  [ct_pktstart] -> we_delay1/1(d)
  [ct_dv] -> we_delay2/1(d)
  we_delay1/1(q) -> pktlen_check/1(pkt_start)
  we_delay2/1(q) -> dv_block_check/1(dv), pktlen_check/2(dv)
  pktlen_check/1(error) -> we_delay7/1(d)
  dv_block_check/1(error) -> we_delay29/1(d)
  [cnt_rst] -> Subsystem6/1(rst)
  we_delay7/1(q) -> [ct_pktlen_err], Subsystem6/2(in0)
  we_delay29/1(q) -> [ct_dvblk_err], Subsystem6/3(in1)
  Subsystem6/1(out0) -> ct_dv_err/1(out_pktlen_err_cnt)
  Subsystem6/2(out1) -> ct_dv_err/2(out_dvblock_err_cnt)
  [cnt_rst] -> Subsystem9/1(rst)
  [ct_bank_error_g0] -> Subsystem9/2(in0)
  [ct_en_sync_error_g0] -> Subsystem9/3(in1)
  [ct_d256] -> Slice43/1
  Slice43/1 -> Relational21/2
  [ct_pktfreq] -> Relational21/1
  Relational21/1 -> Logical16/2
  [ct_dv] -> Delay19/1
  Delay19/1 -> Logical16/1
  Logical16/1 -> [freq_sync_error]
  [cnt_rst] -> Subsystem16/1(rst)
  [freq_sync_error] -> Subsystem16/3(in1)
  [rd_go_err_g] -> Subsystem16/2(in0)
  Subsystem16/1(out0) -> ct_status3/1(out_out_go_err)
  Subsystem16/2(out1) -> ct_status3/2(out_freq_sync_err)
  [cnt_rst] -> Subsystem20/1(rst)
  [ct_en_sync_error_g1] -> Subsystem9/5(in3)
  [ct_bank_error_g1] -> Subsystem9/4(in2)
  Subsystem9/2(out1) -> ct_status0/2(out_err_en_sync0)
  Subsystem9/4(out3) -> ct_status0/4(out_err_en_sync1)
  Subsystem9/1(out0) -> ct_status0/1(out_err_bank0)
  Subsystem9/3(out2) -> ct_status0/3(out_err_bank1)
  [hmc_err_rdrdy_g0] -> Subsystem20/3(in1)
  [hmc_err_wrrdy_g0] -> Subsystem20/2(in0)
  Subsystem20/2(out1) -> ct_status1/2(out_err_wrrdy0)
  Subsystem20/1(out0) -> ct_status1/1(out_err_rdrdy0)
  Subsystem20/4(out3) -> ct_status1/4(out_err_rdrdy1)
  Subsystem20/6(out5) -> ct_status1/6(out_wr_ctr1)
  Subsystem20/5(out4) -> ct_status1/5(out_err_wrrdy1)
  Subsystem20/3(out2) -> ct_status1/3(out_wr_ctr0)
  [wr_en_final_g0] -> Subsystem20/4(in2)
  [hmc_err_wrrdy_g1] -> Subsystem20/5(in3)
  [hmc_err_rdrdy_g1] -> Subsystem20/6(in4)
  [wr_en_final_g1] -> Subsystem20/7(in5)
  [cnt_rst] -> Subsystem21/1(rst)
  [hmc_postokay_g0] -> Inverter/1
  [hmc_init_done_g0] -> Inverter3/1
  [hmc_init_done_g1] -> Inverter5/1
  [hmc_postokay_g1] -> Inverter4/1
  Subsystem21/2(out1) -> ct_status4/2(out_init_err0)
  Subsystem21/4(out3) -> ct_status4/4(out_init_err1)
  Subsystem21/3(out2) -> ct_status4/3(out_post_err1)
  Subsystem21/1(out0) -> ct_status4/1(out_post_err0)
  Inverter/1 -> Subsystem21/2(in0)
  Inverter3/1 -> Subsystem21/3(in1)
  Inverter4/1 -> Subsystem21/4(in2)
  Inverter5/1 -> Subsystem21/5(in3)
  [cnt_rst] -> Subsystem22/1(rst)
  [hmc_dv_clash_g] -> Subsystem22/2(in0)
  [hmc_dv_fixed_clash_g] -> Subsystem22/3(in1)
  [hmc_fifo_full_g] -> Subsystem22/4(in2)
  Subsystem22/3(out2) -> ct_status5/3(out_fifo_full_err)
  Subsystem22/1(out0) -> ct_status5/1(out_dv_clash)
  Subsystem22/2(out1) -> ct_status5/2(out_dv_fixed_clash)
  [cthmc_sync_err_g0] -> Subsystem16/4(in2)
  Subsystem16/3(out2) -> ct_status3/3(out_hmc_sync_error)
  we_delay49/1(q) -> [ct_tag_insert_sel]
  edge_detect2/1(out) -> [ct_rst_err_latch]
  we_delay47/1(q) -> edge_detect2/1(in)
  we_delay48/1(q) -> [ct_fake_data_error]
  we_delay13/1(q) -> [ct_tvg_en]
  we_delay50/1(q) -> [ct_tvg_en2]
  Constant12/1 -> ct_control0/5(sim_5)
  Constant21/1 -> ct_control0/4(sim_4)
  Constant20/1 -> ct_control0/3(sim_3)
  Constant15/1 -> ct_control0/1(sim_1)
  ct_control0/1(in_tvg_en) -> we_delay13/1(d)
  ct_control0/2(in_tvg_en2) -> we_delay50/1(d)
  ct_control0/3(in_rst_err_latch) -> we_delay47/1(d)
  ct_control0/4(in_fake_error) -> we_delay48/1(d)
  ct_control0/5(in_tag_insert) -> we_delay49/1(d)
  we_delay126/1(q) -> [obuf_read_gap]
  ct_control0/6(in_obuf_read_gap) -> we_delay126/1(d)
  Constant30/1 -> ct_control0/6(sim_6)
  we_delay41/1(q) -> [ct_num_xeng]
  we_delay112/1(q) -> [ct_num_xeng_recip]  "NUM_X_RECIP"
  ct_control1/2(in_num_x_recip) -> we_delay112/1(d)
  ct_control1/1(in_num_x) -> we_delay41/1(d)
  we_delay114/1(q) -> [ct_x_per_board]
  ct_control1/3(in_x_per_board) -> we_delay114/1(d)
  we_delay39/1(q) -> [ct_chans_per_x], Slice3/1  "PER_X"
  we_delay113/1(q) -> [ct_chans_per_board]
  ct_control2/1(in_chans_per_x) -> we_delay39/1(d)
  ct_control2/2(in_chans_per_board) -> we_delay113/1(d)
  Slice3/1 -> Slice39/1, [ct_chans_per_x_par]  "PARPAR"
  we_delay115/1(q) -> [ct_x_per_board_recip]
  ct_control1/4(in_x_per_board_recip) -> we_delay115/1(d)
  we_delay38/1(q) -> [ct_num_x_boards]
  ct_control3/1(in_num_x_boards) -> we_delay38/1(d)
  we_delay37/1(q) -> [ct_num_x_boards_recip]
  ct_control3/2(in_num_x_boards_recip) -> we_delay37/1(d)
  ct_control3/3(in_chans_per_x_recip) -> we_delay124/1(d)
  we_delay124/1(q) -> Reinterpret40/1, [ct_chans_per_x_recip]
  Slice39/1 -> [ct_chans_per_x_hmc_par]  "per_x_hmc"
  Reinterpret40/1 -> [ct_chans_per_x_hmc_par_recip]
  Constant49/1 -> ct_control1/1(sim_1)
  Constant53/1 -> ct_control1/2(sim_2)
  Constant33/1 -> ct_control1/3(sim_3)
  Constant23/1 -> ct_control2/1(sim_1)
  Constant50/1 -> ct_control2/2(sim_2)
  Constant54/1 -> ct_control1/4(sim_4)
  Constant32/1 -> ct_control3/1(sim_1)
  Constant14/1 -> ct_control3/2(sim_2)
  Constant44/1 -> ct_control3/3(sim_3)
  Slice18/1 -> [tvgtone_p0]
  Slice19/1 -> [tvgtone_p1]
  [q_dv] -> Subsystem17/1(In1)
  Subsystem17/1(Out1) -> ct_in_dv_rate/1(out_reg)
  Slice36/1 -> we_delay116/1(d)
  Constant38/1 -> ct_control4/1(sim_1)
  ct_control4/1(in_ct_board_offset) -> Slice36/1
  ct_control5/1(in_ct_freq_gen_offset) -> we_delay117/1(d)
  Constant39/1 -> ct_control5/1(sim_1)
  we_delay116/1(q) -> [ct_board_hmc_offset]
  we_delay117/1(q) -> [ct_freq_gen_offset]
  [obuf_proc_err_miss_g] -> Subsystem22/5(in3)
  Subsystem22/4(out3) -> ct_status5/4(out_proc_err_miss)
  [q_sync] -> hmc_ct/1(in_sync)
  hmc_ct/4(pkt_start) -> [ct_pktstart]
  hmc_ct/1(out_sync) -> [ct_sync]
  hmc_ct/2(out_dv) -> [ct_dv]
  hmc_ct/3(out_d256) -> [ct_d256]
  hmc_ct/5(freq_id) -> [ct_pktfreq]
  [q_dv] -> hmc_ct/2(in_dv)
  Concat4/1 -> hmc_ct/3(in_d128), [q_d128]
  hmc_ct/6(x_index) -> [ct_pkt_x_index]
  hmc_ct/7(x_pkt_index) -> [ct_pkt_x_offset]
  [q_d64_0] -> Concat4/1
  [q_d64_1] -> Concat4/2
  pipeline80/1(q) -> [flag_sync]
  pipeline81/1(q) -> [flag_misc]
  pipeline82/1(q) -> [flag_dvalid]
  pipeline83/1(q) -> [flag_time]
  pipeline85/1(q) -> time_gen1/4(rd_sync_in)
  pipeline87/1(q) -> time_gen1/6(rd_misc_in)
  Delay/1 -> pipeline85/1(d)  "gapsync"
  Delay2/1 -> pipeline86/1(d)  "gapdata"
  Mux1/1 -> pipeline87/1(d)  "gapvalid"
  [time80] -> Slice2/1
  pipeline86/1(q) -> time_gen1/5(rd_en)
  time_gen1/1(rd_sync_out) -> pipeline80/1(d)
  time_gen1/4(rd_misc_out) -> pipeline81/1(d)
  time_gen1/2(rd_dvalid) -> pipeline82/1(d)
  time_gen1/3(rd_val_out) -> pipeline83/1(d)
  Slice2/1 -> time_gen1/3(wr_val_in)
  [ct_tvg_en2] -> Mux1/1
  Delay17/1 -> Delay5/1
  Delay6/1 -> Mux1/2
  Delay7/1 -> tvg/1(sync), Delay/1
  Delay18/1 -> Delay7/1
  Delay16/1 -> Delay6/1
  Delay5/1 -> tvg/2(dv), Delay2/1
  tvg/1(data256) -> Mux1/3
  [ct_d256] -> Delay16/1
  [ct_dv] -> Delay17/1
  [ct_sync] -> Delay18/1
  pipeline185/1(q) -> pipeline24/1(d)
  pipeline177/1(q) -> pipeline179/1(d)
  pipeline179/1(q) -> pipeline23/1(d)
  pipeline23/1(q) -> pipeline185/1(d)
  pipeline24/1(q) -> [flag_pktstart]
  pipeline25/1(q) -> pipeline183/1(d)
  pipeline183/1(q) -> pipeline184/1(d)
  pipeline187/1(q) -> pipeline186/1(d)
  pipeline186/1(q) -> [flag_pktfreq]
  pipeline184/1(q) -> pipeline187/1(d)
  pipeline168/1(q) -> pipeline169/1(d)
  pipeline169/1(q) -> pipeline170/1(d)
  pipeline170/1(q) -> pipeline171/1(d)
  pipeline171/1(q) -> pipeline172/1(d)
  pipeline172/1(q) -> [flag_pktxindex]
  pipeline173/1(q) -> pipeline174/1(d)
  pipeline174/1(q) -> pipeline175/1(d)
  pipeline175/1(q) -> pipeline176/1(d)
  pipeline176/1(q) -> pipeline178/1(d)
  pipeline178/1(q) -> [flag_pktxoffset]
  [ct_pkt_x_index] -> Delay15/1
  [ct_pkt_x_offset] -> Delay20/1
  [ct_pktfreq] -> Delay1/1
  [ct_pktstart] -> Delay4/1
  Delay4/1 -> pipeline177/1(d)
  Delay1/1 -> pipeline25/1(d)
  Delay15/1 -> pipeline168/1(d)
  Delay20/1 -> pipeline173/1(d)
  [sync80] -> time_gen1/1(wr_sync_in)
  [valid80] -> time_gen1/2(wr_en)
  [time80_48] -> Subsystem/1(time)
  [sync80] -> Subsystem/2(sync)
  [valid80] -> Subsystem/3(dv)
  Subsystem/1(msw) -> sync_time_msw/1(out_reg)
  Subsystem/2(ls32) -> sync_time_lsw/1(out_reg)
  [flag_pktfreq] -> Subsystem27/3(value)
  [cnt_rst] -> Subsystem27/1(rst)
  [flag_dvalid] -> Subsystem27/2(en)
  Subsystem27/1(current) -> flag_pktfreq_stats/1(out_current)
  Subsystem27/3(min) -> flag_pktfreq_stats/3(out_min)
  Subsystem27/2(max) -> flag_pktfreq_stats/2(out_max)
  [flag_pktxindex] -> Subsystem28/3(value)
  [cnt_rst] -> Subsystem28/1(rst)
  [flag_dvalid] -> Subsystem28/2(en)
  Subsystem28/1(current) -> flag_pktxindex_stats/1(out_current)
  Subsystem28/3(min) -> flag_pktxindex_stats/3(out_min)
  Subsystem28/2(max) -> flag_pktxindex_stats/2(out_max)
  [flag_pktxoffset] -> Subsystem29/3(value)
  [cnt_rst] -> Subsystem29/1(rst)
  [flag_dvalid] -> Subsystem29/2(en)
  Subsystem29/1(current) -> flag_pktxoffset_stats/1(out_current)
  Subsystem29/3(min) -> flag_pktxoffset_stats/3(out_min)
  Subsystem29/2(max) -> flag_pktxoffset_stats/2(out_max)
  [flag_time] -> Subsystem30/3(value)
  [cnt_rst] -> Subsystem30/1(rst)
  [flag_pktstart] -> Subsystem30/2(en)
  Subsystem30/1(current) -> flag_time_stats/1(out_current)
  Subsystem30/3(min) -> flag_time_stats/3(out_min)
  Subsystem30/2(max) -> flag_time_stats/2(out_max)
  Constant22/1 -> ct_control0/2(sim_2)
  Subsystem10/1(out0) -> ct_status2/1(out_addr_err0_cnt)
  Subsystem10/2(out1) -> ct_status2/2(out_sync_cnt)
  Constant16/1 -> [time80_48]
